simulink library "Sattelite_PD_Controller_lib"  (R2016a)
settings: Solver=ode45  StartTime=0.0  StopTime=10.0  RelTol=1e-3
values from neighbouring files (symbols this model uses):
  kd = 2*z*wn    (= 0.068)    [Dynamic_Dependant_control.m]
  kp = wn.^2    [Dynamic_Dependant_control.m]
libraries: Quaternion_Subtraction x1
settings Model: Creator=devantormey  LastModifiedBy=devantormey
settings DataIOCC: LimitDataPoints=on
settings DebuggingCC: AllowSymbolicDim=off

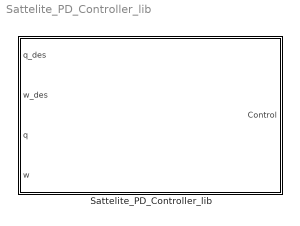
== system Sattelite_PD_Controller_lib ==
  "Sattelite_PD_Controller_lib " : Subsystem

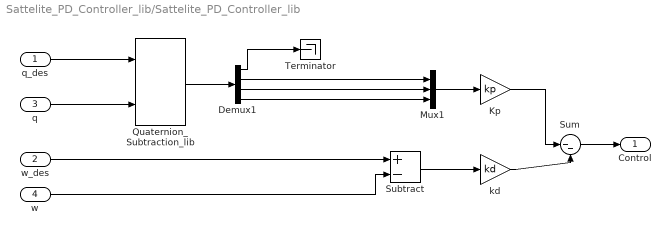
== system Sattelite_PD_Controller_lib/Sattelite_PD_Controller_lib  ==
  q_des : Inport
  "w_des " : Inport  Port=2
  q : Inport  Port=3
  w : Inport  Port=4
  Demux1 : Demux
  Kp : Gain  Gain=kp
  Mux1 : Mux  Inputs=3
  Quaternion_Subtraction_lib : Quaternion_Subtraction/Quaternion_Subtraction_lib
  Subtract : Sum  Inputs=+-
  Sum : Sum  Inputs=|--
  Terminator : Terminator
  kd : Gain  Gain=kd
  Control : Outport
  wires:
  kd/1 -> Sum/2
  Mux1/1 -> Kp/1
  Demux1/4 -> Mux1/3
  Demux1/2 -> Mux1/1
  Demux1/3 -> Mux1/2
  Kp/1 -> Sum/1
  Sum/1 -> Control/1
  Subtract/1 -> kd/1
  "w_des "/1 -> Subtract/1
  w/1 -> Subtract/2
  q_des/1 -> Quaternion_Subtraction_lib/1
  q/1 -> Quaternion_Subtraction_lib/2
  Quaternion_Subtraction_lib/1 -> Demux1/1
  Demux1/1 -> Terminator/1
